simulink model "SystemModelControlled"  (R2015a)
settings: Solver=ode45  StartTime=0.0  StopTime=T  RelTol=1e-3
values from neighbouring files (symbols this model uses):
  A = [3.92291500745 1 0 0 -5.78414696994 0 1 0 3.79889038796 0 0 1 ... (16 elements, 4x4)]    [ssfinal.mat]
  B = [1 0 0 0]    [ssfinal.mat]
  C = [0 0.000180250108713 -0.000200069339657 0]    [ssfinal.mat]
  fs = 100    [codigo_pt2_grupo51.m]
  Nbar = Nu+K*Nx    [codigo_pt2_grupo51.m]
undefined symbols (not defined in the file or in its folder): K, M
settings Model: Creator=Diogo  LastModifiedBy=Diogo

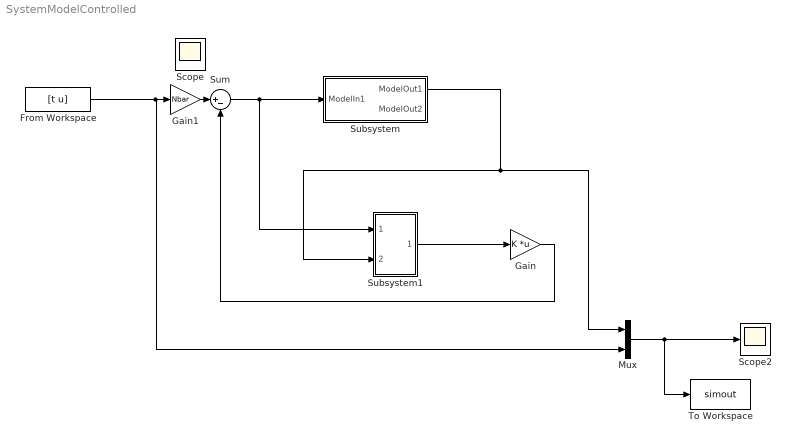
== system SystemModelControlled ==
  From Workspace : FromWorkspace  VariableName=[t u]  SampleTime=1/fs
  Gain : Gain  Gain=K  Multiplication=Matrix(K*u)
  Gain1 : Gain  Gain=Nbar
  Mux : Mux  Inputs=2
  Scope2 : Scope
      settings: SaveName=ScopeData2
  Subsystem : Subsystem
  Subsystem1 : Subsystem
  Sum : Sum  Inputs=|+-
  To Workspace : ToWorkspace  VariableName=simout  SaveFormat=Structure With Time  SampleTime=-1
  Scope : Scope
  wires:
  Sum/1 -> Subsystem1/1(ObsIn1), Subsystem/1(ModelIn1)
  Subsystem/1(ModelOut1) -> Mux/1, Subsystem1/2(ObsIn2)
  Subsystem1/1(ObsOut1) -> Gain/1
  Gain/1 -> Sum/2
  From Workspace/1 -> Gain1/1, Mux/2
  Mux/1 -> To Workspace/1, Scope2/1
  Gain1/1 -> Sum/1

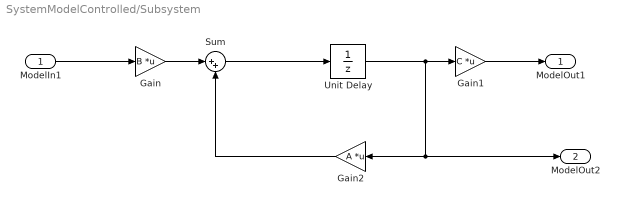
== system SystemModelControlled/Subsystem ==
  ModelIn1 : Inport
  Gain : Gain  Gain=B  Multiplication=Matrix(K*u)
  Gain1 : Gain  Gain=C  Multiplication=Matrix(K*u)
  Gain2 : Gain  Gain=A  Multiplication=Matrix(K*u)
  Sum : Sum  Inputs=|++
  Unit Delay : UnitDelay  SampleTime=-1
  ModelOut1 : Outport
  ModelOut2 : Outport  Port=2
  wires:
  Gain/1 -> Sum/1
  Sum/1 -> Unit Delay/1
  Unit Delay/1 -> Gain2/1, ModelOut2/1, Gain1/1
  Gain2/1 -> Sum/2
  ModelIn1/1 -> Gain/1
  Gain1/1 -> ModelOut1/1

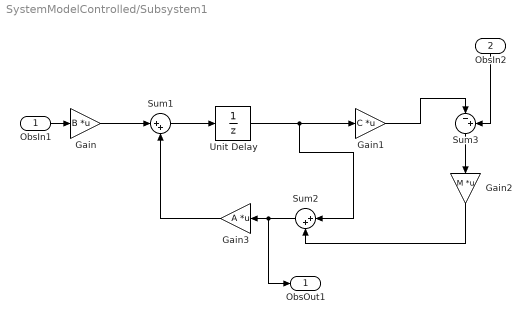
== system SystemModelControlled/Subsystem1 ==
  ObsIn1 : Inport
  ObsIn2 : Inport  Port=2
  Gain : Gain  Gain=B  Multiplication=Matrix(K*u)
  Gain1 : Gain  Gain=C  Multiplication=Matrix(K*u)
  Gain2 : Gain  Gain=M  Multiplication=Matrix(K*u)
  Gain3 : Gain  Gain=A  Multiplication=Matrix(K*u)
  Sum1 : Sum  Inputs=|++
  Sum2 : Sum  Inputs=|++
  Sum3 : Sum  Inputs=|-+
  Unit Delay : UnitDelay  SampleTime=-1
  ObsOut1 : Outport
  wires:
  Sum2/1 -> ObsOut1/1, Gain3/1
  Unit Delay/1 -> Sum2/1, Gain1/1
  Gain3/1 -> Sum1/2
  ObsIn1/1 -> Gain/1
  Sum1/1 -> Unit Delay/1
  Gain2/1 -> Sum2/2
  Sum3/1 -> Gain2/1
  Gain1/1 -> Sum3/1
  ObsIn2/1 -> Sum3/2
  Gain/1 -> Sum1/1
